simulink model "simulink_pwn"  (R2020a)
settings: Solver=VariableStepAuto  StartTime=0.0  StopTime=10.0  RelTol=1e-3
libraries: commsrccod2 x2, dspquant2 x2, commchan3 x1, dsparch4 x1
settings Model: Creator=Administrator  LastModifiedBy=SEELEa317
settings DataIOCC: ReturnWorkspaceOutputs=off
settings DebuggingCC: ArithmeticOperatorsInVariantConditions=warning
settings SFSimCC: CustomCodeUndefinedFunction=UseInterfaceOnly

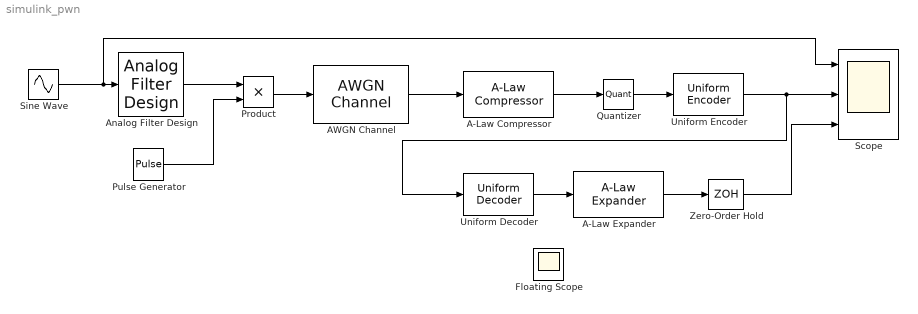
== system simulink_pwn ==
  A-Law Compressor : commsrccod2/A-Law Compressor  A=87.6  V=1
      settings: SourceProductBaseCode=CM
  A-Law Expander : commsrccod2/A-Law Expander  A=87.6  V=20
      settings: SourceProductBaseCode=CM
  AWGN Channel : commchan3/AWGN Channel  InputProcessing=Columns as channels (frame based)  seed=67  noiseMode="Signal to noise ratio  (Eb/No)"  EbNodB=10  EsNodB=10  SNRdB=10  bitsPerSym=1  Ps=1  Tsym=1  variance=1
  Analog Filter Design : dsparch4/Analog Filter Design  method=Butterworth  filttype=Lowpass  N=8  Wlo=30  Whi=80  Rp=2  Rs=40
  Floating Scope : Scope
      settings: Floating=on
  Product : Product
  Pulse Generator : DiscretePulseGenerator  PulseType=Time based  Period=1/32  PulseWidth=5
  Quantizer : Quantizer  QuantizationInterval=1
  Scope : Scope  NumInputPorts=3
  Sine Wave : Sin  Amplitude=128  Frequency=2*pi  SampleTime=0
  Uniform Decoder : dspquant2/Uniform Decoder  peak=20  bits=8  overflowMode=Saturate  otype=Double
      settings: SourceProductBaseCode=DS
  Uniform Encoder : dspquant2/Uniform Encoder  peak=1  bits=8  otype=Unsigned integer
  Zero-Order Hold : ZeroOrderHold  SampleTime=-1
  wires:
  Sine Wave/1 -> Scope/1, Analog Filter Design/1
  Analog Filter Design/1 -> Product/1
  Pulse Generator/1 -> Product/2
  Product/1 -> AWGN Channel/1
  AWGN Channel/1 -> A-Law Compressor/1
  A-Law Compressor/1 -> Quantizer/1
  Quantizer/1 -> Uniform Encoder/1
  Uniform Encoder/1 -> Uniform Decoder/1, Scope/2
  Zero-Order Hold/1 -> Scope/3
  Uniform Decoder/1 -> A-Law Expander/1
  A-Law Expander/1 -> Zero-Order Hold/1
